simulink model "model_State_of_charge_battery"  (R2019a)
settings: Solver=ode45  StartTime=0.0  StopTime=5  RelTol=1e-3  EnableMultiTasking=on
values from neighbouring files (symbols this model uses):
  C1 = 0.003    [Parameters_State_of_charge_battery.m]
  C2 = C1    (= 0.003)    [Parameters_State_of_charge_battery.m]
  freq = 5000    [Parameters_State_of_charge_battery.m]
  highCur = 120    [Parameters_State_of_charge_battery.m]
  highSOC = 95    [Parameters_State_of_charge_battery.m]
  highVolt = 1050    [Parameters_State_of_charge_battery.m]
  initA = 0.88    [Parameters_State_of_charge_battery.m]
  initD = 0.00001    (= 1e-05)    [Parameters_State_of_charge_battery.m]
  L1 = 0.04    [Parameters_State_of_charge_battery.m]
  Lbus = 0.387e-06    (= 3.87e-07)    [Parameters_State_of_charge_battery.m]
  lowCur = -120    [Parameters_State_of_charge_battery.m]
  lowSOC = 65    [Parameters_State_of_charge_battery.m]
  lowVolt = 880    [Parameters_State_of_charge_battery.m]
  NomVoltage = 44.4    [Parameters_State_of_charge_battery.m]
  Rc1 = 0.02    [Parameters_State_of_charge_battery.m]
  Rc2 = Rc1    (= 0.02)    [Parameters_State_of_charge_battery.m]
  stepTime = 0    [Parameters_State_of_charge_battery.m]
  t1 = 0.5/freq    (= 0.0001)    [Parameters_State_of_charge_battery.m]
  t2 = 1/freq    (= 0.0002)    [Parameters_State_of_charge_battery.m]
  Vsource = 1050    [Parameters_State_of_charge_battery.m]
undefined symbols (not defined in the file or in its folder): DMfreq, Ion, Lithium
libraries: electricdrivelib x22, powerlib x18, simulink x8, powerlib_extras x4
settings Model: Creator=axelreds  LastModifiedBy=Dominion
settings DataIOCC: LimitDataPoints=on  SaveFormat=Array  ReturnWorkspaceOutputs=off
settings OptimizationCC: ExpressionDepthLimit=2147483647  LifeSpan=inf
settings DebuggingCC: UnderspecifiedInitializationDetection=Classic  MergeDetectMultiDrivingBlocksExec=none  SolverPrmCheckMsg=warning  StateNameClashWarn=warning  SFUnexpectedBacktrackingDiag=warning  SFNoUnconditionalDefaultTransitionDiag=warning  SFExecutionAtInitializationDiag=none  ArithmeticOperatorsInVariantConditions=warning
settings HardwareCC: ProdBitPerPointer=32  ProdBitPerSizeT=32  ProdBitPerPtrDiffT=32  ProdLargestAtomicFloat=None  ProdIntDivRoundTo=Undefined  ProdEndianess=Unspecified  ProdWordSize=32  ProdHWDeviceType=32-bit Generic
settings ModelReferenceCC: PropagateSignalLabelsOutOfModel=off
settings SFSimCC: SimUseLocalCustomCode=off
settings RTWCC: RTWUseLocalCustomCode=off
settings CodeAppCC: StateflowObjectComments=on
settings GRTTargetCC: TargetLangStandard=C89/C90 (ANSI)  GeneratePreprocessorConditionals=Disable all
settings ConfigComp: CovMetricSettings=dw  CovHtmlReporting=on  CovSaveCumulativeToWorkspaceVar=on  CovSaveSingleToWorkspaceVar=on  CovExternalEMLEnable=off
settings SimscapeCC: SimscapeNormalizeSystem=off

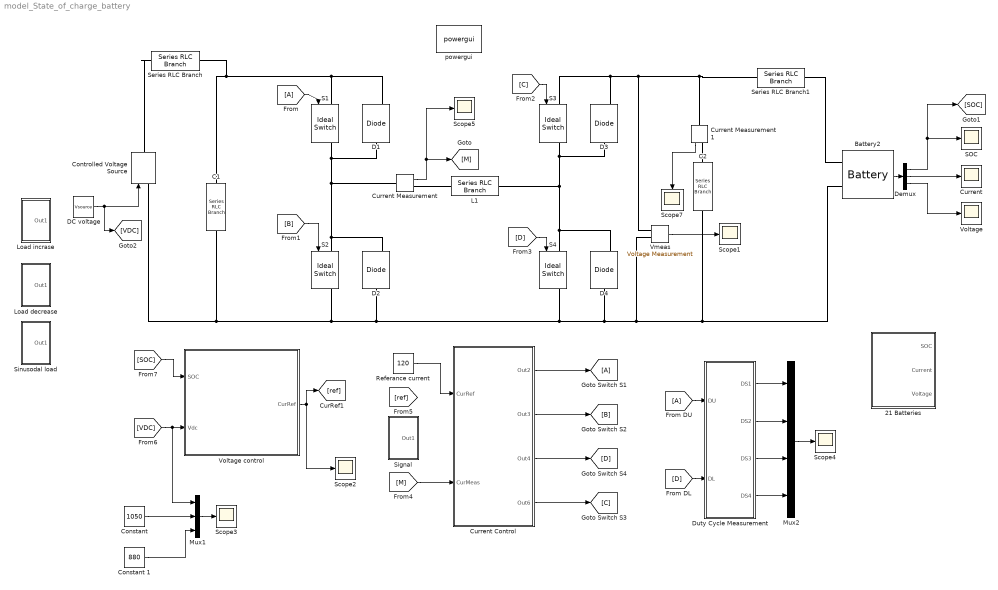
== system model_State_of_charge_battery ==
  21 Batteries : Subsystem
  Battery2 : electricdrivelib/Extra Sources/Battery  BatType=Lithium-Ion  ShowTempParam=off  ThermalPreset=no  ShowAgeParam=off  NomV=21*NomVoltage  NomQ=RatedCap  SOC=inSOC  Batt_Tr=30  PresetModel=on  MaxQ=75  MinV=5.4  FullV=1085.3016  Dis_rate=32.6087  R=0.12432  Normal_OP=67.8261  expZone="[1007.3518      3.6847826]"  current=[50 120 300]  Units=Ampere-hour  Tci=20  NomT=20  T2=-30  MaxQ2=4.8  FullV2=7.1  Normal_OP2=5.655  expZone2="[6.58           1]"  Rca=0.6  ti=2000  Dp=0  Neq0=0  Tsim=1e6  Ta1=25  Qeol=5.4*0.9  Reol=0.013333*1.2  Char_age=[2.3478, 3]  Dis_age=[2.3478, 10]  N1=1500  N2=10500  N3=1000  N4=1400  Ta2=45  N5=950
      settings: SourceProductName=Simscape Electrical
  C1 : powerlib/Elements/Series RLC Branch  LConnTagsString=__new0  RConnTagsString=__new0  BranchType=RC  Resistance=Rc1  Inductance=1e-3  SetiL0=off  InitialCurrent=0  Capacitance=C1  Setx0=on  InitialVoltage=Vc1  Measurements=None
      settings: SourceProductName=Simscape Electrical
  C2 : powerlib/Elements/Series RLC Branch  LConnTagsString=__new0  RConnTagsString=__new0  BranchType=RC  Resistance=Rc2  Inductance=1e-3  SetiL0=off  InitialCurrent=0  Capacitance=C2  Setx0=on  InitialVoltage=Vc2  Measurements=None
      settings: SourceProductName=Simscape Electrical
  "Constant " : Constant  Value=1050
  Constant 1 : Constant  Value=880
  Controlled Voltage Source : powerlib/Electrical Sources/Controlled Voltage Source  Initialize=on  Source_Type=AC  Amplitude=0  Phase=0  Frequency=0  Measurements=None
      settings: SourceProductName=Simscape Electrical
  Current : Scope
  Current Control : Subsystem
  Current Measurement : powerlib/Measurements/Current Measurement  PhasorSimulation=off  OutputType=Complex  PSBequivalent=0
      settings: SourceProductName=Simscape Electrical
  Current Measurement1 : powerlib/Measurements/Current Measurement  PhasorSimulation=off  OutputType=Complex  PSBequivalent=0
      settings: SourceProductName=Simscape Electrical
  D{1..4} (4 alike) : powerlib/Power Electronics/Diode  Ron=0.001  Lon=0  Vf=0.8  IC=0  UseSnubber=off  Rs=500  Cs=250e-9  Measurements=on
      settings: SourceProductName=Simscape Electrical
  DC voltage : Constant  Value=Vsource
  Demux : Demux  Outputs=3
  Duty Cycle Measurement : Subsystem
  L1 : powerlib/Elements/Series RLC Branch  LConnTagsString=__new0  RConnTagsString=__new0  BranchType=L  Resistance=0  Inductance=L1*2  SetiL0=off  InitialCurrent=120  Capacitance=0  Setx0=off  InitialVoltage=0  Measurements=None
      settings: SourceProductName=Simscape Electrical
  Load decrease : Subsystem
  Load incrase : Subsystem
  Mux1 : Mux  Inputs=3
  Mux2 : Mux
  Referance current : Constant  Value=120
  S1 : powerlib/Power Electronics/Ideal Switch  Ron=0.001  Lon=0  IC=0  Rs=1e5  Cs=inf  Measurements=on
      settings: SourceProductName=Simscape Electrical
  S2 : powerlib/Power Electronics/Ideal Switch  Ron=0.001  Lon=0  IC=0  Rs=1e5  Cs=inf  Measurements=on
      settings: SourceProductName=Simscape Electrical
  S3 : powerlib/Power Electronics/Ideal Switch  Ron=0.001  Lon=0  IC=1  Rs=1e5  Cs=inf  Measurements=on
      settings: SourceProductName=Simscape Electrical
  S4 : powerlib/Power Electronics/Ideal Switch  Ron=0.001  Lon=0  IC=0  Rs=1e5  Cs=inf  Measurements=on
      settings: SourceProductName=Simscape Electrical
  SOC : Scope
  Scope{1..5,7} (6 alike) : Scope
  Series RLC Branch : powerlib/Elements/Series RLC Branch  LConnTagsString=__new0  RConnTagsString=__new0  BranchType=L  Resistance=0.05  Inductance=Lbus  SetiL0=off  InitialCurrent=0  Capacitance=1e-6  Setx0=off  InitialVoltage=0  Measurements=None
      settings: SourceProductName=Simscape Electrical
  Series RLC Branch1 : powerlib/Elements/Series RLC Branch  LConnTagsString=__new0  RConnTagsString=__new0  BranchType=L  Resistance=0.0005  Inductance=Lbus  SetiL0=off  InitialCurrent=0  Capacitance=1e-6  Setx0=off  InitialVoltage=0  Measurements=None
      settings: SourceProductName=Simscape Electrical
  Signal : Subsystem
  Sinusodal load : Subsystem
  Vmeas : powerlib/Measurements/Voltage Measurement  PhasorSimulation=off  OutputType=Complex  PSBequivalent=0
      settings: SourceProductName=Simscape Electrical
  Voltage : Scope
  Voltage control : Subsystem
  powergui : powerlib/powergui  Priority=1  SimulationMode=Discrete  SampleTime=50e-6  frequency=60  Iterations=50  frequencyindice=0  Pbase=100e6  ErrMax=1e-4  UnitsV=kV  UnitsW=MW  buscounter=0  FunctionMessages=off  echomessages=off  EnableUseOfTLC=off  CurrentSourceSwitches=off  DisableSnubberDevices=off  DisableRonSwitches=off  DisableVfSwitches=off  DisplayEquations=off  AutomaticDiscreteSolvers=off  SolverType=Tustin  Interpol=off  ExternalGateDelay=off  methode=off  Ts=100  x0status=blocks  SPID=off  SwTol=0  HookPort=off  NonlinearTolerance=0  nMaxIteration=15  ContinueOnMaxIteration=off  RestoreLinks=warning  ResistiveCurrentMeasurement=off  Frange=[0:2:500]  Ylog=off  Xlog=on  ShowGrid=off  save=off  variable=ZData  structure=0  ZoomFFT=off  StartTime=0.0  cycles=1  DisplayStyle=1  fundamental=60  FreqAxis=off  MaxFrequency=1000  frequencyindicesteady=1  RmsSteady=1  display=off
      settings: SourceProductName=Simscape Electrical
  wires:
  Current Measurement/1 -> Scope5/1, [M]
  Vmeas/1 -> Scope1/1
  [B] -> S2/1
  [A] -> S1/1
  [D] -> S4/1
  [C] -> S3/1
  Demux/1 -> [SOC], SOC/1
  Demux/2 -> Current/1
  Demux/3 -> Voltage/1
  [A] -> Duty Cycle Measurement/1(DU)
  [D] -> Duty Cycle Measurement/2(DL)
  Duty Cycle Measurement/1(DS1) -> Mux2/1
  Duty Cycle Measurement/4(DS4) -> Mux2/4
  Duty Cycle Measurement/3(DS3) -> Mux2/3
  Mux2/1 -> Scope4/1
  Duty Cycle Measurement/2(DS2) -> Mux2/2
  Current Measurement1/1 -> Scope7/1
  [SOC] -> Voltage control/1(SOC)
  Voltage control/1(CurRef) -> [ref], Scope2/1
  Current Control/1(Out2) -> [A]
  Current Control/2(Out3) -> [B]
  Current Control/3(Out4) -> [D]
  Current Control/4(Out6) -> [C]
  Referance current/1 -> Current Control/1(CurRef)
  [M] -> Current Control/2(CurMeas)
  "Constant "/1 -> Mux1/2
  Mux1/1 -> Scope3/1
  Constant 1/1 -> Mux1/3
  DC voltage/1 -> [VDC], Controlled Voltage Source/1
  [VDC] -> Mux1/1, Voltage control/2(Vdc)
  Battery2/1 -> Demux/1
  connections:
  S2/LConn1 -- D2/RConn1 -- Current Measurement/LConn1 -- D1/LConn1 -- S1/RConn1
  S2/RConn1 -- Controlled Voltage Source/LConn1 -- C1/RConn1 -- Battery2/LConn2 -- C2/RConn1 -- Vmeas/LConn2 -- D4/LConn1 -- S4/RConn1 -- D2/LConn1
  S4/LConn1 -- D4/RConn1 -- L1/RConn1 -- D3/LConn1 -- S3/RConn1
  S1/LConn1 -- Series RLC Branch/RConn1 -- C1/LConn1 -- D1/RConn1
  S3/LConn1 -- Current Measurement1/LConn1 -- Series RLC Branch1/LConn1 -- Vmeas/LConn1 -- D3/RConn1
  Current Measurement/RConn1 -- L1/LConn1
  Series RLC Branch/LConn1 -- Controlled Voltage Source/RConn1
  Series RLC Branch1/RConn1 -- Battery2/LConn1
  Current Measurement1/RConn1 -- C2/LConn1

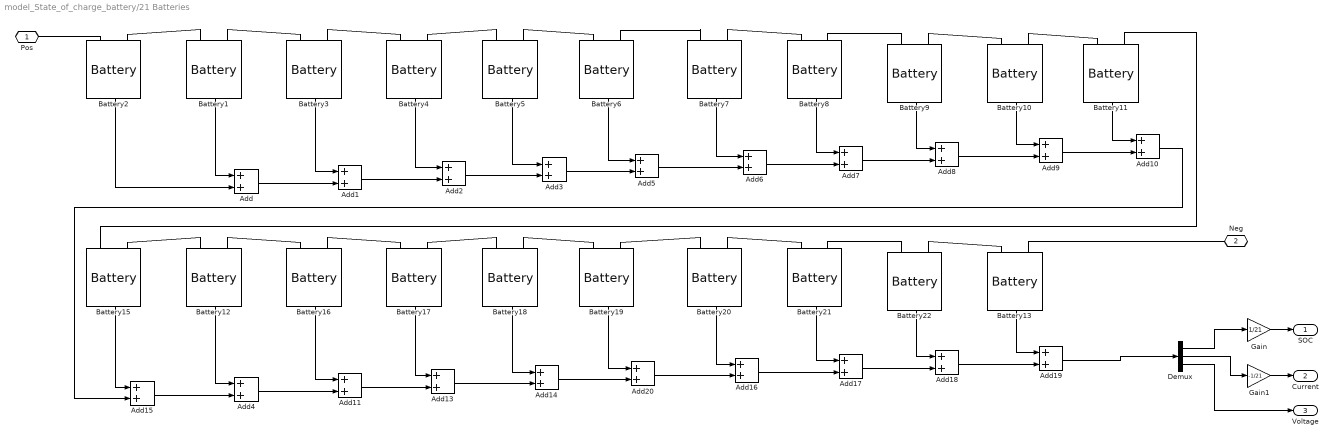
== system model_State_of_charge_battery/21 Batteries ==
  Add{,1..11,13..20} (20 alike) : Sum
  Battery{1..13,16..22} (20 alike) : electricdrivelib/Extra Sources/Battery  BatType=Lithium-Ion  ShowTempParam=off  ThermalPreset=no  ShowAgeParam=off  NomV=NomVoltage  NomQ=RatedCap  SOC=inSOC  Batt_Tr=30  PresetModel=on  MaxQ=75  MinV=5.4  FullV=51.681  Dis_rate=32.6087  R=0.00592  Normal_OP=67.8261  expZone="[47.9691      3.68478]"  current=[50 120 300]  Units=Ampere-hour  Tci=20  NomT=20  T2=-30  MaxQ2=4.8  FullV2=7.1  Normal_OP2=5.655  expZone2="[6.58           1]"  Rca=0.6  ti=2000  Dp=0  Neq0=0  Tsim=1e6  Ta1=25  Qeol=5.4*0.9  Reol=0.013333*1.2  Char_age=[2.3478, 3]  Dis_age=[2.3478, 10]  N1=1500  N2=10500  N3=1000  N4=1400  Ta2=45  N5=950
      settings: SourceProductName=Simscape Electrical
  Battery15 : electricdrivelib/Extra Sources/Battery  BatType=Lithium-Ion  ShowTempParam=off  ThermalPreset=no  ShowAgeParam=off  NomV=NomVoltage  NomQ=RatedCap  SOC=inSOC  Batt_Tr=30  PresetModel=on  MaxQ=75  MinV=5.4  FullV=51.681  Dis_rate=32.6087  R=0.00592  Normal_OP=67.8261  expZone="[47.9691      3.68478]"  current=[50 150 300]  Units=Ampere-hour  Tci=20  NomT=20  T2=-30  MaxQ2=4.8  FullV2=7.1  Normal_OP2=5.655  expZone2="[6.58           1]"  Rca=0.6  ti=2000  Dp=0  Neq0=0  Tsim=1e6  Ta1=25  Qeol=5.4*0.9  Reol=0.013333*1.2  Char_age=[2.3478, 3]  Dis_age=[2.3478, 10]  N1=1500  N2=10500  N3=1000  N4=1400  Ta2=45  N5=950
      settings: SourceProductName=Simscape Electrical
  Demux : Demux  Outputs=3
  Gain : Gain  Gain=1/21
  Gain1 : Gain  Gain=-1/21
  Pos : PMIOPort  Side=Left
  Neg : PMIOPort  Port=2  Side=Left
  SOC : Outport
  Current : Outport  Port=2
  Voltage : Outport  Port=3
  wires:
  Demux/2 -> Gain1/1
  Gain1/1 -> Current/1
  Demux/1 -> Gain/1
  Gain/1 -> SOC/1
  Demux/3 -> Voltage/1
  Battery11/1 -> Add10/1
  Add9/1 -> Add10/2
  Add8/1 -> Add9/2
  Battery10/1 -> Add9/1
  Battery9/1 -> Add8/1
  Add7/1 -> Add8/2
  Battery8/1 -> Add7/1
  Add6/1 -> Add7/2
  Battery7/1 -> Add6/1
  Battery4/1 -> Add2/1
  Add19/1 -> Demux/1
  Add18/1 -> Add19/2
  Battery13/1 -> Add19/1
  Battery22/1 -> Add18/1
  Add17/1 -> Add18/2
  Battery21/1 -> Add17/1
  Add16/1 -> Add17/2
  Battery20/1 -> Add16/1
  Battery16/1 -> Add11/1
  Battery18/1 -> Add14/1
  Battery17/1 -> Add13/1
  Battery19/1 -> Add20/1
  Battery1/1 -> Add/1
  Battery3/1 -> Add1/1
  Battery2/1 -> Add/2
  Add/1 -> Add1/2
  Add1/1 -> Add2/2
  Add2/1 -> Add3/2
  Battery5/1 -> Add3/1
  Add3/1 -> Add5/2
  Battery6/1 -> Add5/1
  Add5/1 -> Add6/2
  Battery12/1 -> Add4/1
  Add11/1 -> Add13/2
  Add13/1 -> Add14/2
  Add14/1 -> Add20/2
  Add20/1 -> Add16/2
  Add10/1 -> Add15/2
  Add4/1 -> Add11/2
  Add15/1 -> Add4/2
  Battery15/1 -> Add15/1
  connections:
  Battery7/LConn1 -- Battery6/LConn2
  Battery9/LConn2 -- Battery10/LConn1
  Battery7/LConn2 -- Battery8/LConn1
  Battery10/LConn2 -- Battery11/LConn1
  Battery9/LConn1 -- Battery8/LConn2
  Battery5/LConn2 -- Battery6/LConn1
  Battery5/LConn1 -- Battery4/LConn2
  Battery3/LConn2 -- Battery4/LConn1
  Battery1/LConn2 -- Battery3/LConn1
  Battery1/LConn1 -- Battery2/LConn2
  Pos/RConn1 -- Battery2/LConn1
  Battery15/LConn1 -- Battery11/LConn2
  Battery18/LConn2 -- Battery19/LConn1
  Battery18/LConn1 -- Battery17/LConn2
  Battery22/LConn1 -- Battery21/LConn2
  Battery22/LConn2 -- Battery13/LConn1
  Battery20/LConn2 -- Battery21/LConn1
  Battery12/LConn2 -- Battery16/LConn1
  Battery13/LConn2 -- Neg/RConn1
  Battery20/LConn1 -- Battery19/LConn2
  Battery12/LConn1 -- Battery15/LConn2
  Battery16/LConn2 -- Battery17/LConn1

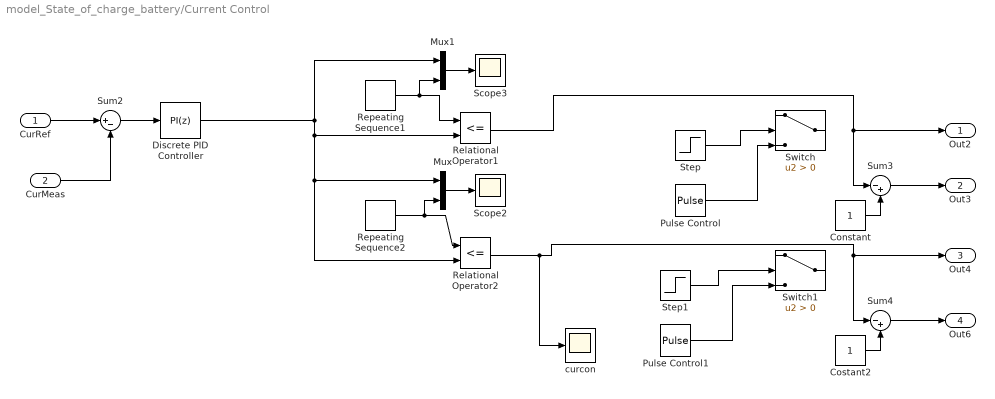
== system model_State_of_charge_battery/Current Control ==
  CurRef : Inport
  CurMeas : Inport  Port=2
  Constant : Constant
  Costant2 : Constant
  Discrete PID Controller : simulink/Continuous/PID Controller  Controller=PI  Form=Parallel  TimeDomain=Discrete-time  SampleTime=2/freq  IntegratorMethod=Forward Euler  FilterMethod=Forward Euler  ControllerParametersSource=internal  P=2/120  I=10/120  D=0  UseFilter=on  N=100  TunerSelectOption=Transfer Function Based (PID Tuner App)  InitialConditionSource=internal  InitialConditionForIntegrator=0  InitialConditionForFilter=0  DifferentiatorICPrevScaledInput=0  ExternalReset=none  TrackingMode=off  Kt=1  LimitOutput=off  UpperSaturationLimit=inf  LowerSaturationLimit=-inf  LinearizeAsGain=off  AntiWindupMode=none  Kb=1  POutMin=[]  POutMax=[]  IOutMin=[]  IOutMax=[]  DOutMin=[]  DOutMax=[]  NOutMin=[]  NOutMax=[]  SumOutMin=[]  SumOutMax=[]  SaturationOutMin=[]  SaturationOutMax=[]  PParamMin=[]  PParamMax=[]  IParamMin=[]  IParamMax=[]  DParamMin=[]  DParamMax=[]  NParamMin=[]  NParamMax=[]  KbParamMin=[]  KbParamMax=[]  KtParamMin=[]  KtParamMax=[]  KbOutMin=[]  KbOutMax=[]  KtOutMin=[]  KtOutMax=[]  IntegratorOutMin=[]  IntegratorOutMax=[]  FilterOutMin=[]  FilterOutMax=[]  SumI1OutMin=[]  SumI1OutMax=[]  SumI2OutMin=[]  SumI2OutMax=[]  SumI3OutMin=[]  SumI3OutMax=[]  SumI4OutMin=[]  SumI4OutMax=[]  SumDOutMin=[]  SumDOutMax=[]  DifferentiatorOutMin=[]  DifferentiatorOutMax=[]  FilterDiffOutCoefMin=[]  FilterDiffOutCoefMax=[]  ReciprocalOutMin=[]  ReciprocalOutMax=[]  SumDenOutMin=[]  SumDenOutMax=[]  SumNumOutMin=[]  SumNumOutMax=[]  DivideOutMin=[]  DivideOutMax=[]  IntegratorContinuousStateAttributes=''  IntegratorStateMustResolveToSignalObject=off  IntegratorRTWStateStorageClass=Auto  FilterContinuousStateAttributes=''  FilterStateMustResolveToSignalObject=off  FilterRTWStateStorageClass=Auto  ParallelPVariant=InternalParameters  IdealPVariant=Disabled  IVariant=InternalParameters  DVariant=Disabled  IntegratorVariant=Discrete  SatVariant=Disabled  AWVariant=Passthrough  PCopyVariant=Disabled  TRVariant=Disabled  FdbkBlocksVariant=Forward  IdealPFdbkVariant=Disabled  SatFdbkVariant=Disabled  DerivativeFilterVariant=Disabled  NVariant=Disabled  NCopyVariant=Disabled_SignalSpec  FilterICVariant=Disabled  IntegratorICVariant=InternalICs  ExternalResetVariant=Disabled  TRSumVariant=Passthrough  SumFdbkVariant=Disabled  SumVariant=Sum_PI
  Mux : Mux  Inputs=2
  Mux1 : Mux  Inputs=2
  Pulse Control : DiscretePulseGenerator  PulseType=Time based  Period=1/freq  PulseWidth=initA
  Pulse Control1 : DiscretePulseGenerator  PulseType=Time based  Period=1/freq  PulseWidth=initD
  Relational Operator1 : RelationalOperator  Operator=<=  OutDataTypeStr=boolean  RndMeth=Nearest
  Relational Operator2 : RelationalOperator  Operator=<=  OutDataTypeStr=boolean  RndMeth=Nearest
  Repeating Sequence1 : simulink/Sources/Repeating Sequence  rep_seq_t=[0 t1 t2]  rep_seq_y=[-1 0 -1]
  Repeating Sequence2 : simulink/Sources/Repeating Sequence  rep_seq_t=[0 t1 t2]  rep_seq_y=[0 1 0]
  Scope2 : Scope
  Scope3 : Scope
  Step : Step  Time=stepTime  Before=-1  SampleTime=0
  Step1 : Step  Time=stepTime  Before=-1  SampleTime=0
  Sum2 : Sum  Inputs=|+-
  Sum3 : Sum  Inputs=|-+
  Sum4 : Sum  Inputs=|-+
  Switch : Switch  Criteria=u2 > Threshold
  Switch1 : Switch  Criteria=u2 > Threshold
  curcon : Scope
  Out2 : Outport
  Out3 : Outport  Port=2
  Out4 : Outport  Port=3
  Out6 : Outport  Port=4
  wires:
  CurRef/1 -> Sum2/1
  Relational Operator1/1 -> Out2/1, Sum3/1
  Relational Operator2/1 -> curcon/1, Sum4/1, Out4/1
  Pulse Control1/1 -> Switch1/3
  Sum2/1 -> Discrete PID Controller/1
  Pulse Control/1 -> Switch/3
  Step1/1 -> Switch1/2
  CurMeas/1 -> Sum2/2
  Constant/1 -> Sum3/2
  Sum3/1 -> Out3/1
  Costant2/1 -> Sum4/2
  Sum4/1 -> Out6/1
  Repeating Sequence2/1 -> Mux/2, Relational Operator2/1
  Mux/1 -> Scope2/1
  Repeating Sequence1/1 -> Mux1/2, Relational Operator1/1
  Discrete PID Controller/1 -> Mux/1, Relational Operator2/2, Relational Operator1/2, Mux1/1
  Step/1 -> Switch/2
  Mux1/1 -> Scope3/1

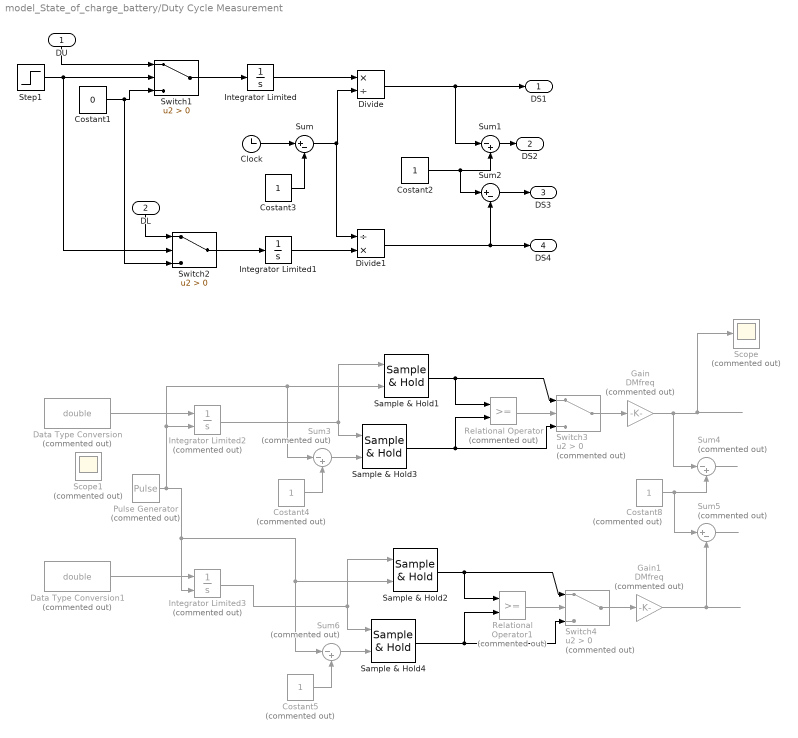
== system model_State_of_charge_battery/Duty Cycle Measurement ==
  DU : Inport
  DL : Inport  Port=2
  Clock : Clock
  Costant1 : Constant  Value=0
  Costant2 : Constant
  Costant3 : Constant
  Costant4 : Constant  Commented=on
  Costant5 : Constant  Commented=on
  Costant8 : Constant  Commented=on
  Data Type Conversion : DataTypeConversion  Commented=on  OutDataTypeStr=double
  Data Type Conversion1 : DataTypeConversion  Commented=on  OutDataTypeStr=double
  Divide : Product  Inputs=*/
  Divide1 : Product  Inputs=/*
  Gain : Gain  Commented=on  Gain=DMfreq
  Gain1 : Gain  Commented=on  Gain=DMfreq
  Integrator Limited : Integrator  UpperSaturationLimit=1  LowerSaturationLimit=0
  Integrator Limited1 : Integrator  UpperSaturationLimit=1  LowerSaturationLimit=0
  Integrator Limited2 : Integrator  Commented=on  ExternalReset=either  UpperSaturationLimit=1  LowerSaturationLimit=0
  Integrator Limited3 : Integrator  Commented=on  ExternalReset=either  UpperSaturationLimit=1  LowerSaturationLimit=0
  Pulse Generator : DiscretePulseGenerator  Commented=on  PulseType=Time based  Period=2/DMfreq  PulseWidth=50
  Relational Operator : RelationalOperator  Commented=on  OutDataTypeStr=boolean  RndMeth=Nearest
  Relational Operator1 : RelationalOperator  Commented=on  OutDataTypeStr=boolean  RndMeth=Nearest
  Sample & Hold{1..4} (4 alike) : powerlib_extras/Control  Blocks/Sample & Hold  ic=0
      settings: SourceProductName=Simscape Electrical  SourceProductBaseCode=PS
  Scope : Scope  Commented=on
  Scope1 : Scope  Commented=on
  Step1 : Step  Before=-1  SampleTime=0
  Sum : Sum  Inputs=|+-
  Sum1 : Sum  Inputs=|-+
  Sum2 : Sum  Inputs=|+-
  Sum3 : Sum  Commented=on  Inputs=|-+
  Sum4 : Sum  Commented=on  Inputs=|-+
  Sum5 : Sum  Commented=on  Inputs=|+-
  Sum6 : Sum  Commented=on  Inputs=|-+
  Switch1 : Switch  Criteria=u2 > Threshold
  Switch2 : Switch  Criteria=u2 > Threshold
  Switch3 : Switch  Commented=on  Criteria=u2 > Threshold
  Switch4 : Switch  Commented=on  Criteria=u2 > Threshold
  DS1 : Outport
  DS2 : Outport  Port=2
  DS3 : Outport  Port=3
  DS4 : Outport  Port=4
  wires:
  Step1/1 -> Switch2/2, Switch1/2
  Costant3/1 -> Sum/2
  Divide/1 -> DS1/1, Sum1/1
  Switch1/1 -> Integrator Limited/1
  Costant1/1 -> Switch2/3, Switch1/3
  Sum/1 -> Divide1/1, Divide/2
  Integrator Limited/1 -> Divide/1
  Clock/1 -> Sum/1
  DU/1 -> Switch1/1
  DL/1 -> Switch2/1
  Switch2/1 -> Integrator Limited1/1
  Integrator Limited1/1 -> Divide1/2
  Divide1/1 -> Sum2/2, DS4/1
  Costant2/1 -> Sum2/1, Sum1/2
  Sum1/1 -> DS2/1
  Sum2/1 -> DS3/1
  ? -> Scope1/1, Data Type Conversion/1
  Gain/1 -> Sum4/1, Scope/1
  Costant8/1 -> Sum5/1, Sum4/2
  Sum4/1 -> ?
  ? -> Data Type Conversion1/1
  Data Type Conversion1/1 -> Integrator Limited3/1
  Data Type Conversion/1 -> Integrator Limited2/1
  Integrator Limited2/1 -> Sample & Hold1/1, Sample & Hold3/1
  Sum5/1 -> ?
  Gain1/1 -> Sum5/2
  Costant4/1 -> Sum3/2
  Sum3/1 -> Sample & Hold3/2
  Sample & Hold3/1 -> Relational Operator/2, Switch3/3
  Sample & Hold1/1 -> Switch3/1, Relational Operator/1
  Relational Operator/1 -> Switch3/2
  Switch3/1 -> Gain/1
  Integrator Limited3/1 -> Sample & Hold2/1, Sample & Hold4/1
  Pulse Generator/1 -> Sum6/1, Sample & Hold2/2, Integrator Limited3/2, Sample & Hold1/2, Sum3/1, Integrator Limited2/2
  Costant5/1 -> Sum6/2
  Sum6/1 -> Sample & Hold4/2
  Sample & Hold4/1 -> Switch4/3, Relational Operator1/2
  Sample & Hold2/1 -> Relational Operator1/1, Switch4/1
  Relational Operator1/1 -> Switch4/2
  Switch4/1 -> Gain1/1

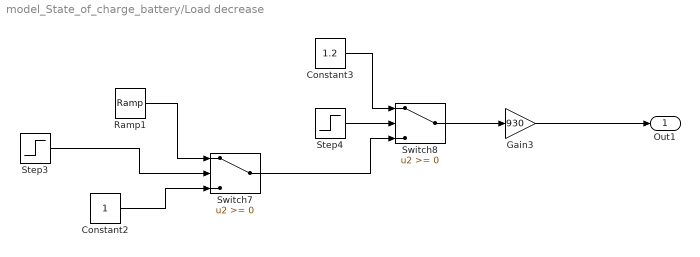
== system model_State_of_charge_battery/Load decrease ==
  Constant2 : Constant
  Constant3 : Constant  Value=1.2
  Gain3 : Gain  Gain=930
  Ramp1 : simulink/Sources/Ramp  slope=0.2/2  start=2  InitialOutput=1
  Step3 : Step  Time=2  Before=-1  SampleTime=0
  Step4 : Step  Time=4  Before=-1  SampleTime=0
  Switch7 : Switch
  Switch8 : Switch
  Out1 : Outport
  wires:
  Gain3/1 -> Out1/1
  Ramp1/1 -> Switch7/1
  Switch7/1 -> Switch8/3
  Constant2/1 -> Switch7/3
  Switch8/1 -> Gain3/1
  Step4/1 -> Switch8/2
  Constant3/1 -> Switch8/1
  Step3/1 -> Switch7/2

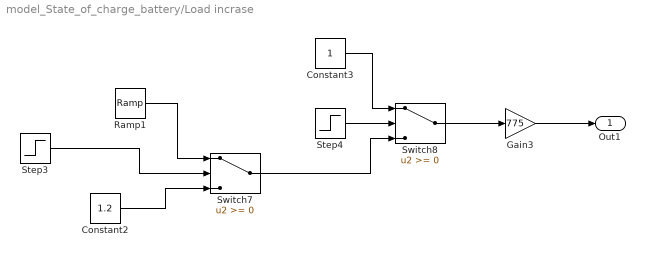
== system model_State_of_charge_battery/Load incrase ==
  Constant2 : Constant  Value=1.2
  Constant3 : Constant
  Gain3 : Gain  Gain=775
  Ramp1 : simulink/Sources/Ramp  slope=-0.2/2  start=2  InitialOutput=1.2
  Step3 : Step  Time=2  Before=-1  SampleTime=0
  Step4 : Step  Time=4  Before=-1  SampleTime=0
  Switch7 : Switch
  Switch8 : Switch
  Out1 : Outport
  wires:
  Ramp1/1 -> Switch7/1
  Switch7/1 -> Switch8/3
  Constant2/1 -> Switch7/3
  Switch8/1 -> Gain3/1
  Step4/1 -> Switch8/2
  Constant3/1 -> Switch8/1
  Step3/1 -> Switch7/2
  Gain3/1 -> Out1/1

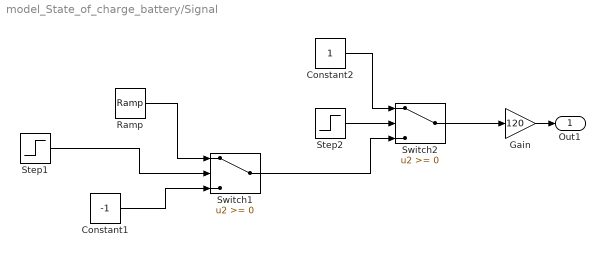
== system model_State_of_charge_battery/Signal ==
  Constant1 : Constant  Value=-1
  Constant2 : Constant
  Gain : Gain  Gain=120
  Ramp : simulink/Sources/Ramp  slope=1  start=2  InitialOutput=-1
  Step1 : Step  Time=2  Before=-1  SampleTime=0
  Step2 : Step  Time=4  Before=-1  SampleTime=0
  Switch1 : Switch
  Switch2 : Switch
  Out1 : Outport
  wires:
  Gain/1 -> Out1/1
  Step1/1 -> Switch1/2
  Constant2/1 -> Switch2/1
  Step2/1 -> Switch2/2
  Switch2/1 -> Gain/1
  Constant1/1 -> Switch1/3
  Switch1/1 -> Switch2/3
  Ramp/1 -> Switch1/1

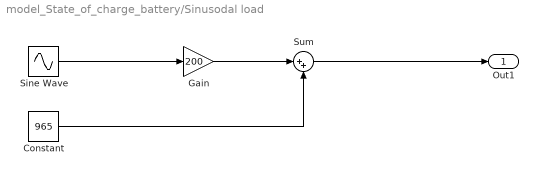
== system model_State_of_charge_battery/Sinusodal load ==
  Constant : Constant  Value=965
  Gain : Gain  Gain=200
  Sine Wave : Sin  Frequency=0.8  SampleTime=0
  Sum : Sum  Inputs=|++
  Out1 : Outport
  wires:
  Constant/1 -> Sum/2
  Sum/1 -> Out1/1
  Gain/1 -> Sum/1
  Sine Wave/1 -> Gain/1

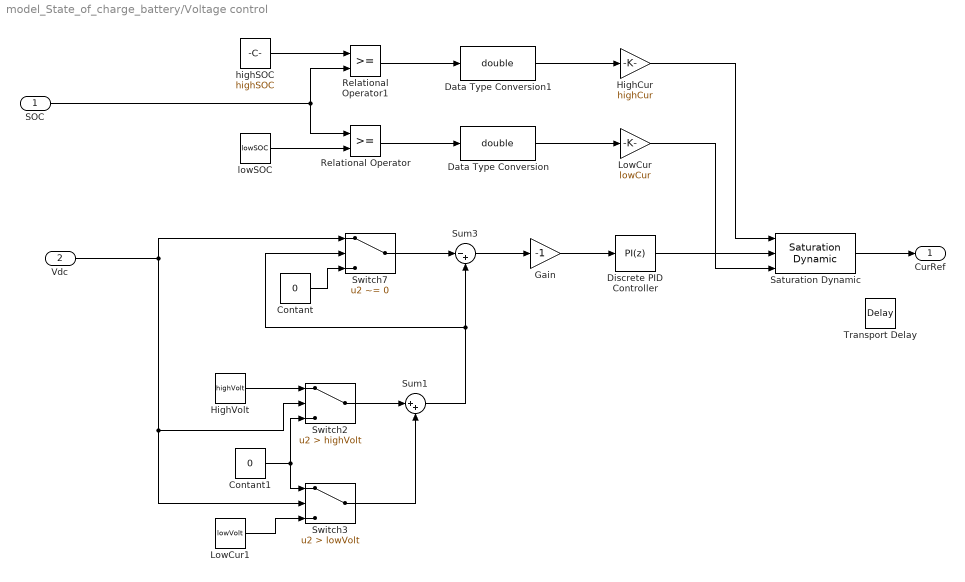
== system model_State_of_charge_battery/Voltage control ==
  SOC : Inport
  Vdc : Inport  Port=2
  Contant : Constant  Value=0
  Contant1 : Constant  Value=0
  Data Type Conversion : DataTypeConversion  OutDataTypeStr=double
  Data Type Conversion1 : DataTypeConversion  OutDataTypeStr=double
  Discrete PID Controller : simulink/Continuous/PID Controller  Controller=PI  Form=Parallel  TimeDomain=Discrete-time  SampleTime=10/freq  IntegratorMethod=Forward Euler  FilterMethod=Forward Euler  ControllerParametersSource=internal  P=0.005  I=1  D=0  UseFilter=on  N=100  TunerSelectOption=Transfer Function Based (PID Tuner App)  InitialConditionSource=internal  InitialConditionForIntegrator=0  InitialConditionForFilter=0  DifferentiatorICPrevScaledInput=0  ExternalReset=none  TrackingMode=off  Kt=1  LimitOutput=off  UpperSaturationLimit=inf  LowerSaturationLimit=-inf  LinearizeAsGain=off  AntiWindupMode=none  Kb=1  POutMin=[]  POutMax=[]  IOutMin=[]  IOutMax=[]  DOutMin=[]  DOutMax=[]  NOutMin=[]  NOutMax=[]  SumOutMin=[]  SumOutMax=[]  SaturationOutMin=[]  SaturationOutMax=[]  PParamMin=[]  PParamMax=[]  IParamMin=[]  IParamMax=[]  DParamMin=[]  DParamMax=[]  NParamMin=[]  NParamMax=[]  KbParamMin=[]  KbParamMax=[]  KtParamMin=[]  KtParamMax=[]  KbOutMin=[]  KbOutMax=[]  KtOutMin=[]  KtOutMax=[]  IntegratorOutMin=[]  IntegratorOutMax=[]  FilterOutMin=[]  FilterOutMax=[]  SumI1OutMin=[]  SumI1OutMax=[]  SumI2OutMin=[]  SumI2OutMax=[]  SumI3OutMin=[]  SumI3OutMax=[]  SumI4OutMin=[]  SumI4OutMax=[]  SumDOutMin=[]  SumDOutMax=[]  DifferentiatorOutMin=[]  DifferentiatorOutMax=[]  FilterDiffOutCoefMin=[]  FilterDiffOutCoefMax=[]  ReciprocalOutMin=[]  ReciprocalOutMax=[]  SumDenOutMin=[]  SumDenOutMax=[]  SumNumOutMin=[]  SumNumOutMax=[]  DivideOutMin=[]  DivideOutMax=[]  IntegratorContinuousStateAttributes=''  IntegratorStateMustResolveToSignalObject=off  IntegratorRTWStateStorageClass=Auto  FilterContinuousStateAttributes=''  FilterStateMustResolveToSignalObject=off  FilterRTWStateStorageClass=Auto  ParallelPVariant=InternalParameters  IdealPVariant=Disabled  IVariant=InternalParameters  DVariant=Disabled  IntegratorVariant=Discrete  SatVariant=Disabled  AWVariant=Passthrough  PCopyVariant=Disabled  TRVariant=Disabled  FdbkBlocksVariant=Forward  IdealPFdbkVariant=Disabled  SatFdbkVariant=Disabled  DerivativeFilterVariant=Disabled  NVariant=Disabled  NCopyVariant=Disabled_SignalSpec  FilterICVariant=Disabled  IntegratorICVariant=InternalICs  ExternalResetVariant=Disabled  TRSumVariant=Passthrough  SumFdbkVariant=Disabled  SumVariant=Sum_PI
  Gain : Gain  Gain=-1
  HighCur : Gain  Gain=highCur
  HighVolt : Constant  Value=highVolt
  LowCur : Gain  Gain=lowCur
  LowCur1 : Constant  Value=lowVolt
  Relational Operator : RelationalOperator  OutDataTypeStr=boolean  RndMeth=Nearest
  Relational Operator1 : RelationalOperator  OutDataTypeStr=boolean  RndMeth=Nearest
  Saturation Dynamic : simulink/Discontinuities/Saturation Dynamic  OutMin=[]  OutMax=[]  OutDataTypeStr=Inherit: Same as second input  OutDataType=fixdt(1, 16)  OutScaling=2^-10  DoSatur=off
  Sum1 : Sum  Inputs=|++
  Sum3 : Sum  Inputs=|-+
  Switch2 : Switch  Criteria=u2 > Threshold  Threshold=highVolt
  Switch3 : Switch  Criteria=u2 > Threshold  Threshold=lowVolt
  Switch7 : Switch  Criteria=u2 ~= 0  Threshold=lowVolt
  Transport Delay : TransportDelay  DelayTime=1/5000
  highSOC : Constant  Value=highSOC
  lowSOC : Constant  Value=lowSOC
  CurRef : Outport
  wires:
  highSOC/1 -> Relational Operator1/1
  lowSOC/1 -> Relational Operator/2
  SOC/1 -> Relational Operator/1, Relational Operator1/2
  Discrete PID Controller/1 -> Saturation Dynamic/2
  HighVolt/1 -> Switch2/1
  LowCur1/1 -> Switch3/3
  Switch2/1 -> Sum1/1
  Switch3/1 -> Sum1/2
  Vdc/1 -> Switch7/1, Switch3/2, Switch2/2
  Sum1/1 -> Switch7/2, Sum3/2
  Sum3/1 -> Gain/1
  Gain/1 -> Discrete PID Controller/1
  HighCur/1 -> Saturation Dynamic/1
  LowCur/1 -> Saturation Dynamic/3
  Contant1/1 -> Switch2/3, Switch3/1
  Relational Operator/1 -> Data Type Conversion/1
  Data Type Conversion/1 -> LowCur/1
  Relational Operator1/1 -> Data Type Conversion1/1
  Data Type Conversion1/1 -> HighCur/1
  Contant/1 -> Switch7/3
  Switch7/1 -> Sum3/1
  Saturation Dynamic/1 -> CurRef/1
